simulink model "hw6_problem8"  (R2016a)
settings: Solver=VariableStepAuto  StartTime=-.01  StopTime=.2  RelTol=1e-3
values from neighbouring files (symbols this model uses):
  f_sw = 10e3    (= 10000)    [hw6.m]
  idr = -(lambda_pm/(2*L)) + sqrt((lambda_pm/(2*L)))^2-((t3ph/((3*P/4)*lambda_pm))^2)    [hw6.m]
  iqr = t3ph/((3*P/4)*lambda_pm)    (= 14.8148148148)    [hw6.m]
  K_id = 0    [hw6.m]
  K_iq = 0    [hw6.m]
  K_pd = 8    [hw6.m]
  K_pq = 5    [hw6.m]
  L = 2e-3    (= 0.002)    [hw6.m]
  lambda_pm = .3    (= 0.3)    [hw6.m]
  P = 6    [hw6.m]
  R = .15    (= 0.15)    [hw6.m]
  Vbus = 500    [hw6.m]
  wre = (P/2)*wr    (= 785.398163397)    [hw6.m]
libraries: dspsigops x3
settings Model: Creator=Seth Barger  LastModifiedBy=Seth Barger

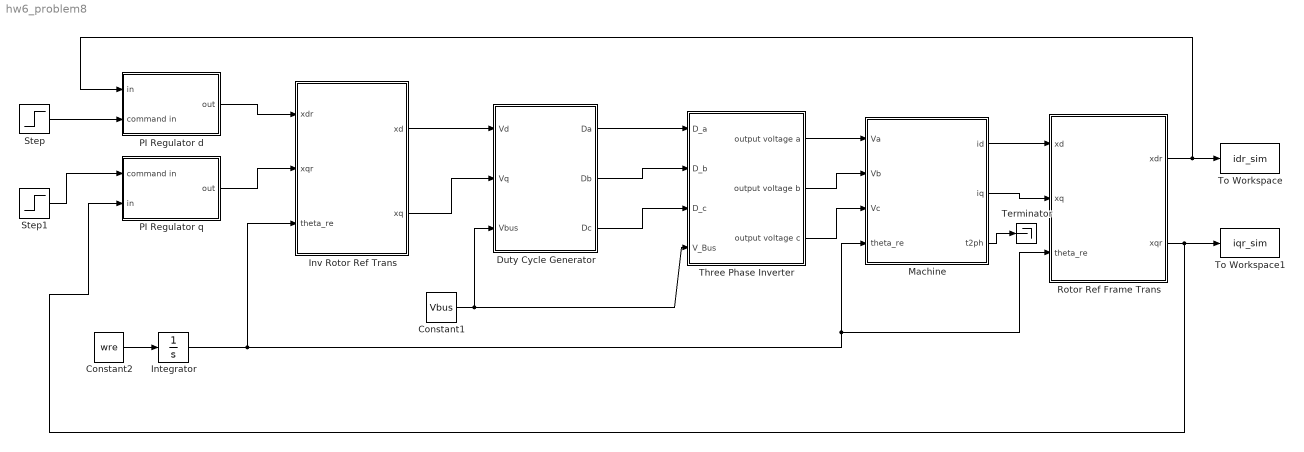
== system hw6_problem8 ==
  Constant1 : Constant  Value=Vbus
  Constant2 : Constant  Value=wre
  Duty Cycle Generator : Subsystem
  Integrator : Integrator
  Inv Rotor Ref Trans : Subsystem
  Machine : Subsystem
  PI Regulator d : Subsystem
  PI Regulator q : Subsystem
  Rotor Ref Frame Trans : Subsystem
  Step : Step  Time=0  After=idr  SampleTime=0
  Step1 : Step  Time=0  After=iqr  SampleTime=0
  Terminator : Terminator
  Three Phase Inverter : Subsystem
  To Workspace : ToWorkspace  VariableName=idr_sim  SampleTime=-1
  To Workspace1 : ToWorkspace  VariableName=iqr_sim  SampleTime=-1
  wires:
  Machine/1(id) -> Rotor Ref Frame Trans/1(xd)
  Machine/2(iq) -> Rotor Ref Frame Trans/2(xq)
  Three Phase Inverter/1(output voltage a) -> Machine/1(Va)
  Three Phase Inverter/2(output voltage b) -> Machine/2(Vb)
  Three Phase Inverter/3(output voltage c) -> Machine/3("Vc ")
  Constant1/1 -> Duty Cycle Generator/3(Vbus), Three Phase Inverter/4(V_Bus)
  Duty Cycle Generator/1(Da) -> Three Phase Inverter/1(D_a)
  Duty Cycle Generator/2(Db) -> Three Phase Inverter/2(D_b)
  Duty Cycle Generator/3(Dc) -> Three Phase Inverter/3(D_c)
  Inv Rotor Ref Trans/1(xd) -> Duty Cycle Generator/1(Vd)
  Inv Rotor Ref Trans/2(xq) -> Duty Cycle Generator/2(Vq)
  Constant2/1 -> Integrator/1
  Integrator/1 -> Inv Rotor Ref Trans/3(theta_re), Rotor Ref Frame Trans/3(theta_re), Machine/4(theta_re)
  Step/1 -> PI Regulator d/2(command in)
  Step1/1 -> PI Regulator q/1(command in)
  Rotor Ref Frame Trans/1(xdr) -> PI Regulator d/1(in), To Workspace/1
  Rotor Ref Frame Trans/2(xqr) -> PI Regulator q/2(in), To Workspace1/1
  PI Regulator q/1(out) -> Inv Rotor Ref Trans/2(xqr)
  PI Regulator d/1(out) -> Inv Rotor Ref Trans/1(xdr)
  Machine/3(t2ph) -> Terminator/1

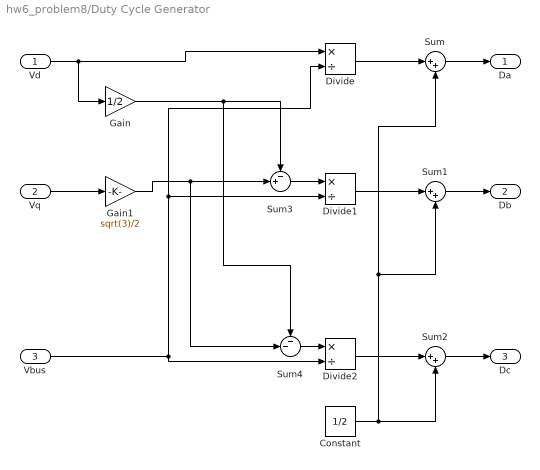
== system hw6_problem8/Duty Cycle Generator ==
  Vd : Inport
  Vq : Inport  Port=2
  Vbus : Inport  Port=3
  Constant : Constant  Value=1/2
  Divide : Product  Inputs=*/
  Divide1 : Product  Inputs=*/
  Divide2 : Product  Inputs=*/
  Gain : Gain  Gain=1/2
  Gain1 : Gain  Gain=sqrt(3)/2
  Sum : Sum  Inputs=|++
  Sum1 : Sum  Inputs=|++
  Sum2 : Sum  Inputs=|++
  Sum3 : Sum  Inputs=-+|
  Sum4 : Sum  Inputs=--|
  Da : Outport
  Db : Outport  Port=2
  Dc : Outport  Port=3
  wires:
  Sum2/1 -> Dc/1
  Constant/1 -> Sum2/2, Sum1/2, Sum/2
  Vd/1 -> Gain/1, Divide/1
  Sum/1 -> Da/1
  Divide1/1 -> Sum1/1
  Sum1/1 -> Db/1
  Vbus/1 -> Divide1/2, Divide/2, Divide2/2
  Vq/1 -> Gain1/1
  Sum3/1 -> Divide1/1
  Gain1/1 -> Sum4/2, Sum3/2
  Sum4/1 -> Divide2/1
  Divide/1 -> Sum/1
  Divide2/1 -> Sum2/1
  Gain/1 -> Sum4/1, Sum3/1

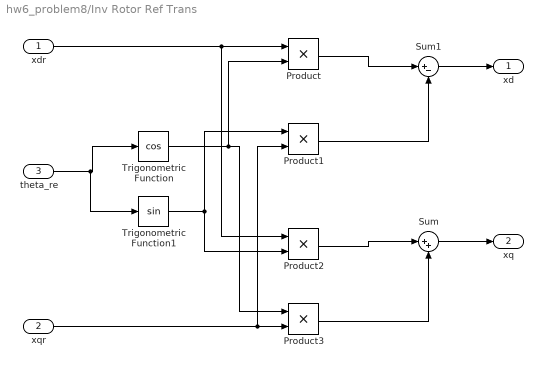
== system hw6_problem8/Inv Rotor Ref Trans ==
  xdr : Inport
  xqr : Inport  Port=2
  theta_re : Inport  Port=3
  Product{,1..3} (4 alike) : Product
  Sum : Sum  Inputs=|++
  Sum1 : Sum  Inputs=|+-
  Trigonometric Function : Trigonometry  Operator=cos
  Trigonometric Function1 : Trigonometry
  xd : Outport
  xq : Outport  Port=2
  wires:
  Product3/1 -> Sum/2
  theta_re/1 -> Trigonometric Function1/1, Trigonometric Function/1
  Product/1 -> Sum1/1
  Sum/1 -> xq/1
  Trigonometric Function/1 -> Product3/1, Product/2
  Product2/1 -> Sum/1
  Sum1/1 -> xd/1
  xqr/1 -> Product3/2, Product1/2
  Product1/1 -> Sum1/2
  xdr/1 -> Product2/1, Product/1
  Trigonometric Function1/1 -> Product2/2, Product1/1

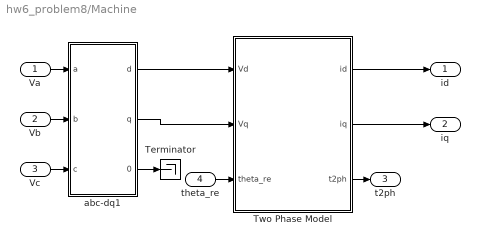
== system hw6_problem8/Machine ==
  Va : Inport
  Vb : Inport  Port=2
  "Vc " : Inport  Port=3
  theta_re : Inport  Port=4
  Terminator : Terminator
  Two Phase Model : Subsystem
  abc-dq1 : Subsystem
  id : Outport
  iq : Outport  Port=2
  t2ph : Outport  Port=3
  wires:
  Two Phase Model/2(iq) -> iq/1
  Vb/1 -> abc-dq1/2(b)
  "Vc "/1 -> abc-dq1/3(c)
  theta_re/1 -> Two Phase Model/3(theta_re)
  Two Phase Model/3(t2ph) -> t2ph/1
  Va/1 -> abc-dq1/1(a)
  abc-dq1/3(0) -> Terminator/1
  abc-dq1/1(d) -> Two Phase Model/1(Vd)
  abc-dq1/2(q) -> Two Phase Model/2(Vq)
  Two Phase Model/1(id) -> id/1

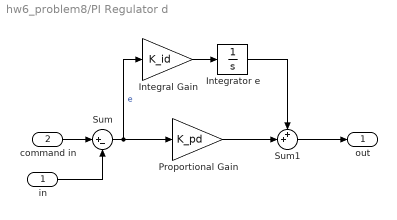
== system hw6_problem8/PI Regulator d ==
  in : Inport
  command in : Inport  Port=2
  Integral Gain : Gain  Gain=K_id  SaturateOnIntegerOverflow=on  OutDataTypeStr=Inherit: Same as input  ParamDataTypeStr=Inherit: Same as input
  Integrator e : Integrator
  Proportional Gain : Gain  Gain=K_pd  SaturateOnIntegerOverflow=on  OutDataTypeStr=Inherit: Same as input  ParamDataTypeStr=Inherit: Same as input
  Sum : Sum  Inputs=|+-  SaturateOnIntegerOverflow=on
  Sum1 : Sum  Inputs=++|  SaturateOnIntegerOverflow=on
  out : Outport
  wires:
  Sum/1 -> Integral Gain/1, Proportional Gain/1  "e"
  command in/1 -> Sum/1
  in/1 -> Sum/2
  Proportional Gain/1 -> Sum1/2
  Sum1/1 -> out/1
  Integral Gain/1 -> Integrator e/1
  Integrator e/1 -> Sum1/1

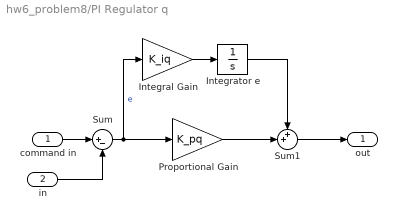
== system hw6_problem8/PI Regulator q ==
  command in : Inport
  in : Inport  Port=2
  Integral Gain : Gain  Gain=K_iq  SaturateOnIntegerOverflow=on  OutDataTypeStr=Inherit: Same as input  ParamDataTypeStr=Inherit: Same as input
  Integrator e : Integrator
  Proportional Gain : Gain  Gain=K_pq  SaturateOnIntegerOverflow=on  OutDataTypeStr=Inherit: Same as input  ParamDataTypeStr=Inherit: Same as input
  Sum : Sum  Inputs=|+-  SaturateOnIntegerOverflow=on
  Sum1 : Sum  Inputs=++|  SaturateOnIntegerOverflow=on
  out : Outport
  wires:
  Sum/1 -> Integral Gain/1, Proportional Gain/1  "e"
  command in/1 -> Sum/1
  in/1 -> Sum/2
  Proportional Gain/1 -> Sum1/2
  Sum1/1 -> out/1
  Integral Gain/1 -> Integrator e/1
  Integrator e/1 -> Sum1/1

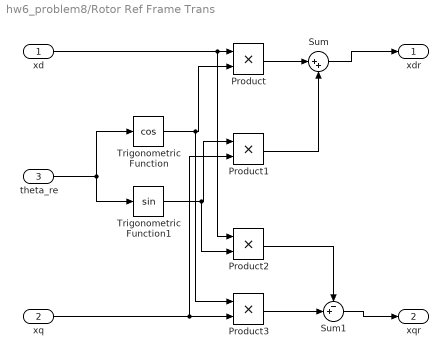
== system hw6_problem8/Rotor Ref Frame Trans ==
  xd : Inport
  xq : Inport  Port=2
  theta_re : Inport  Port=3
  Product{,1..3} (4 alike) : Product
  Sum : Sum  Inputs=|++
  Sum1 : Sum  Inputs=-+|
  Trigonometric Function : Trigonometry  Operator=cos
  Trigonometric Function1 : Trigonometry
  xdr : Outport
  xqr : Outport  Port=2
  wires:
  Product2/1 -> Sum1/1
  Sum/1 -> xdr/1
  Product/1 -> Sum/1
  Product3/1 -> Sum1/2
  Trigonometric Function/1 -> Product3/1, Product/2
  Sum1/1 -> xqr/1
  xq/1 -> Product3/2, Product1/2
  Product1/1 -> Sum/2
  theta_re/1 -> Trigonometric Function/1, Trigonometric Function1/1
  Trigonometric Function1/1 -> Product2/2, Product1/1
  xd/1 -> Product2/1, Product/1

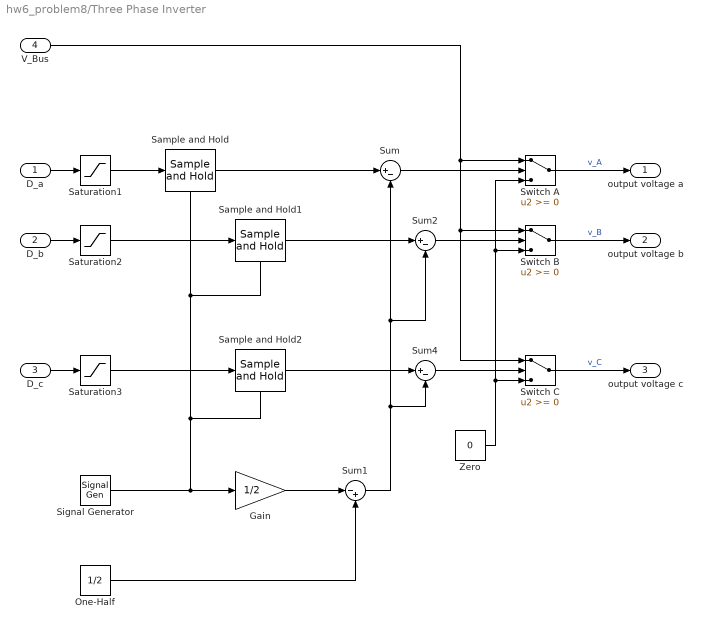
== system hw6_problem8/Three Phase Inverter ==
  D_a : Inport
  D_b : Inport  Port=2
  D_c : Inport  Port=3
  V_Bus : Inport  Port=4
  Gain : Gain  Gain=1/2  SaturateOnIntegerOverflow=on  OutDataTypeStr=Inherit: Same as input  ParamDataTypeStr=Inherit: Same as input
  One-Half : Constant  Value=1/2
  Sample and Hold : dspsigops/Sample and Hold  trig=Falling edge  initCond=0  latchinput=off
  Sample and Hold1 : dspsigops/Sample and Hold  trig=Falling edge  initCond=0  latchinput=off
  Sample and Hold2 : dspsigops/Sample and Hold  trig=Falling edge  initCond=0  latchinput=off
  Saturation1 : Saturate  UpperLimit=1  LowerLimit=0
  Saturation2 : Saturate  UpperLimit=1  LowerLimit=0
  Saturation3 : Saturate  UpperLimit=1  LowerLimit=0
  Signal Generator : SignalGenerator  WaveForm=sawtooth  Frequency=f_sw
  Sum : Sum  Inputs=|+-  SaturateOnIntegerOverflow=on
  Sum1 : Sum  Inputs=|-+  SaturateOnIntegerOverflow=on
  Sum2 : Sum  Inputs=|+-  SaturateOnIntegerOverflow=on
  Sum4 : Sum  Inputs=|+-  SaturateOnIntegerOverflow=on
  Switch A : Switch  SaturateOnIntegerOverflow=on
  Switch B : Switch  SaturateOnIntegerOverflow=on
  Switch C : Switch  SaturateOnIntegerOverflow=on
  Zero : Constant  Value=0
  output voltage a : Outport
  output voltage b : Outport  Port=2
  output voltage c : Outport  Port=3
  wires:
  Sum/1 -> Switch A/2
  Zero/1 -> Switch B/3, Switch A/3, Switch C/3
  Signal Generator/1 -> Sample and Hold/Trigger, Sample and Hold1/Trigger, Sample and Hold2/Trigger, Gain/1
  Gain/1 -> Sum1/1
  One-Half/1 -> Sum1/2
  Sum2/1 -> Switch B/2
  Sum1/1 -> Sum4/2, Sum2/2, Sum/2
  V_Bus/1 -> Switch A/1, Switch B/1, Switch C/1
  D_a/1 -> Saturation1/1
  Sample and Hold/1 -> Sum/1
  D_b/1 -> Saturation2/1
  Sample and Hold1/1 -> Sum2/1
  Saturation1/1 -> Sample and Hold/1
  Saturation2/1 -> Sample and Hold1/1
  D_c/1 -> Saturation3/1
  Saturation3/1 -> Sample and Hold2/1
  Sample and Hold2/1 -> Sum4/1
  Sum4/1 -> Switch C/2
  Switch A/1 -> output voltage a/1  "v_A"
  Switch C/1 -> output voltage c/1  "v_C"
  Switch B/1 -> output voltage b/1  "v_B"

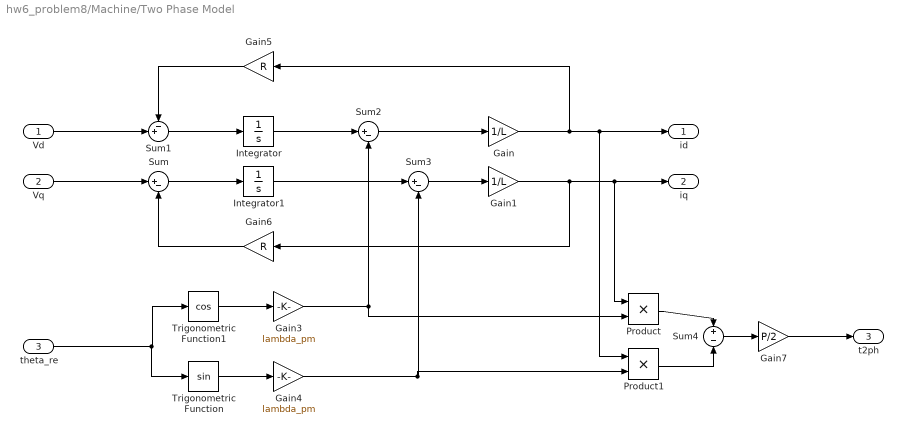
== system hw6_problem8/Machine/Two Phase Model ==
  Vd : Inport
  Vq : Inport  Port=2
  theta_re : Inport  Port=3
  Gain : Gain  Gain=1/L
  Gain1 : Gain  Gain=1/L
  Gain3 : Gain  Gain=lambda_pm
  Gain4 : Gain  Gain=lambda_pm
  Gain5 : Gain  Gain=R
  Gain6 : Gain  Gain=R
  Gain7 : Gain  Gain=P/2
  Integrator : Integrator
  Integrator1 : Integrator
  Product : Product
  Product1 : Product
  Sum : Sum  Inputs=|+-
  Sum1 : Sum  Inputs=-+|
  Sum2 : Sum  Inputs=|+-
  Sum3 : Sum  Inputs=|+-
  Sum4 : Sum  Inputs=+|-
  Trigonometric Function : Trigonometry
  Trigonometric Function1 : Trigonometry  Operator=cos
  id : Outport
  iq : Outport  Port=2
  t2ph : Outport  Port=3
  wires:
  Sum1/1 -> Integrator/1
  Sum4/1 -> Gain7/1
  Integrator/1 -> Sum2/1
  Sum/1 -> Integrator1/1
  Sum3/1 -> Gain1/1
  Product/1 -> Sum4/1
  theta_re/1 -> Trigonometric Function/1, Trigonometric Function1/1
  Trigonometric Function1/1 -> Gain3/1
  Gain4/1 -> Product1/2, Sum3/2
  Sum2/1 -> Gain/1
  Product1/1 -> Sum4/2
  Integrator1/1 -> Sum3/1
  Gain7/1 -> t2ph/1
  Gain1/1 -> Gain6/1, iq/1, Product/1
  Trigonometric Function/1 -> Gain4/1
  Gain/1 -> id/1, Product1/1, Gain5/1
  Gain3/1 -> Sum2/2, Product/2
  Gain6/1 -> Sum/2
  Vq/1 -> Sum/1
  Gain5/1 -> Sum1/1
  Vd/1 -> Sum1/2

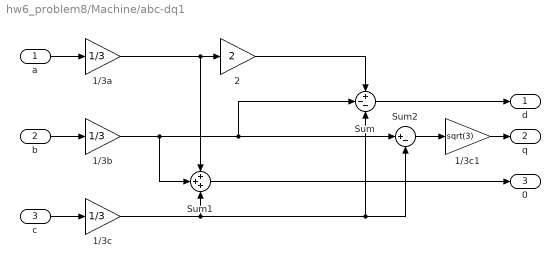
== system hw6_problem8/Machine/abc-dq1 ==
  a : Inport
  b : Inport  Port=2
  c : Inport  Port=3
  1/3a : Gain  Gain=1/3
  1/3b : Gain  Gain=1/3
  1/3c : Gain  Gain=1/3
  1/3c1 : Gain  Gain=sqrt(3)
  2 : Gain  Gain=2
  Sum : Sum  Inputs=+--
  Sum1 : Sum  Inputs=+++
  Sum2 : Sum  Inputs=|+-
  d : Outport
  q : Outport  Port=2
  0 : Outport  Port=3
  wires:
  1/3c1/1 -> q/1
  Sum2/1 -> 1/3c1/1
  Sum1/1 -> 0/1
  1/3c/1 -> Sum/3, Sum2/2, Sum1/3
  Sum/1 -> d/1
  1/3b/1 -> Sum/2, Sum2/1, Sum1/2
  2/1 -> Sum/1
  1/3a/1 -> 2/1, Sum1/1
  a/1 -> 1/3a/1
  b/1 -> 1/3b/1
  c/1 -> 1/3c/1
